simulink library "csu_ctp_coarse_thruster_pulse_command_lib"  (R2014b)
settings: Solver=ode113  StartTime=0.0  StopTime=10.0  RelTol=1e-3
values from neighbouring files (symbols this model uses):
  cac_acs_minimum_coarse_thruster_ontime = 30    [csc_cac_coarse_acs_ctrl_init.m]
  cac_acs_time_gain_x = 20.0    (= 20)    [csc_cac_coarse_acs_ctrl_init.m]
  cac_acs_time_gain_y = 20.0    (= 20)    [csc_cac_coarse_acs_ctrl_init.m]
  cac_acs_time_gain_z = 20.0    (= 20)    [csc_cac_coarse_acs_ctrl_init.m]
  cac_saturation_axial_force = 0*cac_coarse_thruster_force*cosd(15)+4*cac_coarse_thruster_force    [csc_cac_coarse_acs_ctrl_prep.m]
undefined symbols (not defined in the file or in its folder): cac_num_variable, cac_thr_control, cac_thruster_alloc_pad_coarse_x_tq_full_on, cac_thruster_alloc_pad_coarse_x_tq_variable, cac_thruster_alloc_pad_coarse_y_tq_full_on, cac_thruster_alloc_pad_coarse_y_tq_variable, cac_trq_control
libraries: simulink x1
settings Model: Creator=Jim Kaidy  LastModifiedBy=mstewart

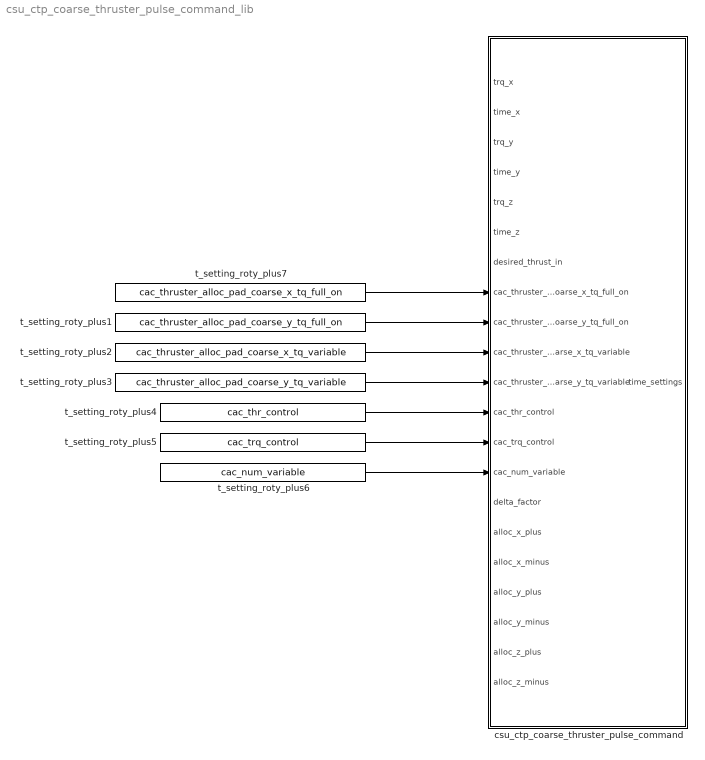
== system csu_ctp_coarse_thruster_pulse_command_lib ==
  csu_ctp_coarse_thruster_pulse_command : Subsystem  TreatAsAtomicUnit=on
  t_setting_roty_plus1 : Constant  Value=cac_thruster_alloc_pad_coarse_y_tq_full_on
  t_setting_roty_plus2 : Constant  Value=cac_thruster_alloc_pad_coarse_x_tq_variable
  t_setting_roty_plus3 : Constant  Value=cac_thruster_alloc_pad_coarse_y_tq_variable
  t_setting_roty_plus4 : Constant  Value=cac_thr_control
  t_setting_roty_plus5 : Constant  Value=cac_trq_control
  t_setting_roty_plus6 : Constant  Value=cac_num_variable
  t_setting_roty_plus7 : Constant  Value=cac_thruster_alloc_pad_coarse_x_tq_full_on
  wires:
  t_setting_roty_plus7/1 -> csu_ctp_coarse_thruster_pulse_command/8(cac_thruster_alloc_pad_coarse_x_tq_full_on)
  t_setting_roty_plus1/1 -> csu_ctp_coarse_thruster_pulse_command/9(cac_thruster_alloc_pad_coarse_y_tq_full_on)
  t_setting_roty_plus2/1 -> csu_ctp_coarse_thruster_pulse_command/10(cac_thruster_alloc_pad_coarse_x_tq_variable)
  t_setting_roty_plus3/1 -> csu_ctp_coarse_thruster_pulse_command/11(cac_thruster_alloc_pad_coarse_y_tq_variable)
  t_setting_roty_plus4/1 -> csu_ctp_coarse_thruster_pulse_command/12(cac_thr_control)
  t_setting_roty_plus5/1 -> csu_ctp_coarse_thruster_pulse_command/13(cac_trq_control)
  t_setting_roty_plus6/1 -> csu_ctp_coarse_thruster_pulse_command/14(cac_num_variable)
  ? -> csu_ctp_coarse_thruster_pulse_command/15(delta_factor)
  ? -> csu_ctp_coarse_thruster_pulse_command/16(alloc_x_plus)
  ? -> csu_ctp_coarse_thruster_pulse_command/17(alloc_x_minus)
  ? -> csu_ctp_coarse_thruster_pulse_command/18(alloc_y_plus)
  ? -> csu_ctp_coarse_thruster_pulse_command/19(alloc_y_minus)
  ? -> csu_ctp_coarse_thruster_pulse_command/20(alloc_z_plus)
  ? -> csu_ctp_coarse_thruster_pulse_command/21(alloc_z_minus)

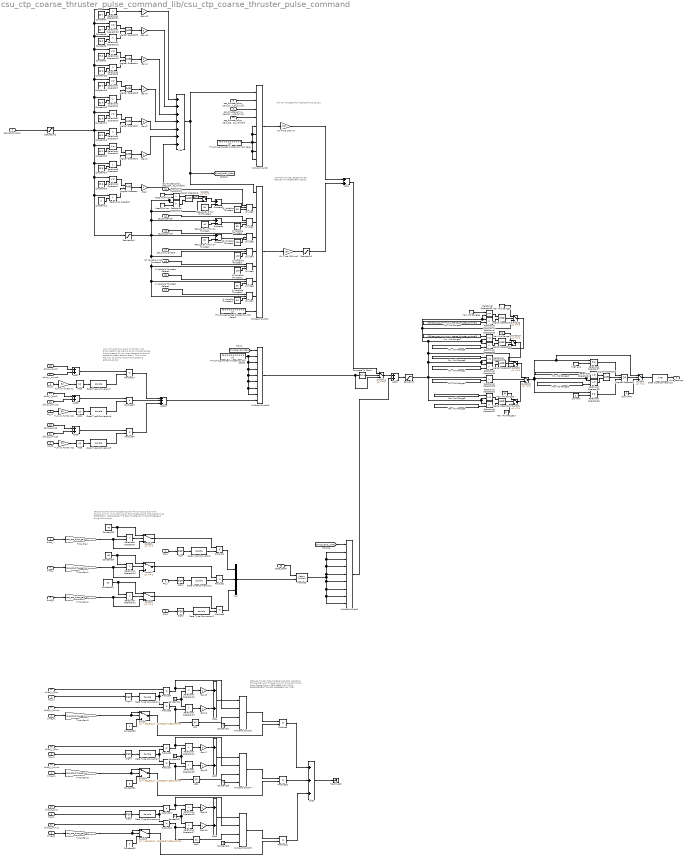
== system csu_ctp_coarse_thruster_pulse_command_lib/csu_ctp_coarse_thruster_pulse_command ==
  note: Attitude Control WItout Descent Control -Coasting
      | Torque Sign and Torque Axis On Time Command
      | From Phase Plane - REPLACED WITH PAIR
      | ENFORCEMENT ON FOR DIFFERENTIAL
      | TIME
  note: Attitude Control With Descent Control Firing
      | Torque Sign and Torque Axis On TIme Command
      | From Phase Plane With Delta Time Offset Matrix (delta_factor)
      | To Bias Thruster On Times Of Descent Firing Commands
  note: Full On Thrusters For Highest Thrust Levels
  note: Variable Thruster Selections For
      |  Desired Thrust Between Levels
  note: ACS with enforcing pairs on for 50 ms
      | to allow delta time logic to allow smaller
      | torque times instead of just when descent
      | control of coarse thrusters asks for them.
      | This is now the way to control biprop and
      | coasting attitude control
  trq_x : Inport
  time_x : Inport  Port=2
  trq_y : Inport  Port=3
  time_y : Inport  Port=4
  trq_z : Inport  Port=5
  time_z : Inport  Port=6
  desired_thrust_in : Inport  Port=7
  cac_thruster_alloc_pad_coarse_x_tq_full_on : Inport  Port=8
  cac_thruster_alloc_pad_coarse_y_tq_full_on : Inport  Port=9
  cac_thruster_alloc_pad_coarse_x_tq_variable : Inport  Port=10
  cac_thruster_alloc_pad_coarse_y_tq_variable : Inport  Port=11
  cac_thr_control : Inport  Port=12
  cac_trq_control : Inport  Port=13
  cac_num_variable : Inport  Port=14
  delta_factor : Inport  Port=15
  alloc_x_plus : Inport  Port=16
  alloc_x_minus : Inport  Port=17
  alloc_y_plus : Inport  Port=18
  alloc_y_minus : Inport  Port=19
  alloc_z_plus : Inport  Port=20
  alloc_z_minus : Inport  Port=21
  "   " : Constant  Value=120
  10 Variable Axial Thrusters1 : InportShadow  Port=13
  10 Variable Thrusters : Constant  Value=100
  10 Variable Thrusters1 : Constant  Value=100
  12 Variable Thrusters : Constant  Value=120
  6 Variable Thrusters : Constant  Value=60
  6 Variable Thrusters Select1 : InportShadow  Port=11
  6 Variable Thrusters1 : Constant  Value=60
  8 Variable Thrusters : Constant  Value=80
  8 Variable Thrusters Select1 : InportShadow  Port=12
  8 Variable Thrusters1 : Constant  Value=80
  Abs{,1..5} (6 alike) : Abs
  Add : Sum  Inputs=+++++++
  Add{1..2,4..9} (8 alike) : Sum
  Add10 : Sum  Inputs=+++
  Add3 : Sum  Inputs=+++
  Compare To Zero1 : simulink/Logic and Bit Operations/Compare To Zero  relop===  OutDataTypeStr=boolean
  Constant1 : Constant  Value=75.2
  Constant{12,21..22,25..28,30..32} (10 alike) : Constant  Value=0
  Constant13 : Constant  Value=23.6
  Constant14 : Constant  Value=23.6
  Constant15 : Constant  Value=42.1
  Constant16 : Constant  Value=42.1
  Constant17 : Constant  Value=51.6
  Constant18 : Constant  Value=51.6
  Constant19 : Constant  Value=65.6
  Constant2 : Constant  Value=75.2
  Constant20 : Constant  Value=65.6
  Constant23 : Constant  Value=40
  Constant24 : Constant  Value=80
  Constant29 : Constant  Value=20
  Constant3 : Constant  Value=93.7
  Constant4 : Constant  Value=93.7
  Data Type Conversion{,1..2,4..9} (9 alike) : DataTypeConversion  OutDataTypeStr=double
  Data Type Conversion3 : DataTypeConversion  OutDataTypeStr=uint8
  Divide{1..7} (7 alike) : Product  Inputs=**/
  Don't Fire : Constant  Value=0
  Gain{,6,8,10} (4 alike) : Gain
  Gain{1,5,7,9} (4 alike) : Gain  Gain=2
  Gain11 : Gain  Gain=6
  Gain12 : Gain  Gain=7
  Gain2 : Gain  Gain=3
  Gain3 : Gain  Gain=4
  Gain4 : Gain  Gain=5
  High end : Constant  Value=100
  Keep Out High : Constant  Value=120
  Keep Out Low : Constant  Value=102
  Logical Operator{,1..7,9..12} (12 alike) : Logic  AllPortsSameDT=off  OutDataTypeStr=boolean
  Logical Operator8 : Logic  Operator=OR  Inputs=3  AllPortsSameDT=off  OutDataTypeStr=boolean
  Low end : Constant  Value=0
  Max Mid Range1 : Constant  Value=70
  Max Mid Range10 : Constant  Value=0
  Max Mid Range2 : Constant  Value=100
  Max Mid Range3 : Constant  Value=cac_acs_minimum_coarse_thruster_ontime
  Max Mid Range4 : Constant  Value=30
  Max Mid Range5 : Constant  Value=cac_acs_minimum_coarse_thruster_ontime
  Max Mid Range6 : Constant  Value=100
  Max Mid Range9 : Constant  Value=cac_acs_minimum_coarse_thruster_ontime/2
  Min  Mid Range1 : Constant  Value=cac_acs_minimum_coarse_thruster_ontime
  Min  Mid Range3 : Constant  Value=100-cac_acs_minimum_coarse_thruster_ontime
  Min  Mid Range4 : Constant  Value=cac_acs_minimum_coarse_thruster_ontime
  Min  Mid Range5 : Constant  Value=100-cac_acs_minimum_coarse_thruster_ontime/2
  Min  Mid Range6 : Constant  Value=100-cac_acs_minimum_coarse_thruster_ontime
  Min  Mid Range7 : Constant  Value=100-cac_acs_minimum_coarse_thruster_ontime/2
  Min  Mid Range8 : Constant  Value=100-cac_acs_minimum_coarse_thruster_ontime
  Multiport Switch{,1..2,6} (4 alike) : MultiPortSwitch  DataPortOrder=Specify indices  Inputs=5  DataPortIndices={7,6,5,4,3,2,1,0}
  Multiport Switch3 : MultiPortSwitch  DataPortOrder=Specify indices  Inputs=5  DataPortIndices={2,1,0}
  Multiport Switch4 : MultiPortSwitch  DataPortOrder=Specify indices  Inputs=5  DataPortIndices={2,1,0}
  Multiport Switch5 : MultiPortSwitch  DataPortOrder=Specify indices  Inputs=5  DataPortIndices={2,1,0}
  Mux : Mux  Inputs=3
  On Time 100 ms : Gain  Gain=100
  On Time 100 ms2 : Gain  Gain=100
  Product{1..4,6..16} (15 alike) : Product
  Product5 : Product  Multiplication=Matrix(*)  RndMeth=Zero
  "Reduce By 2 Full On Thrusters " : Constant  Value=20
  "Reduce By 4 Full On Thrusters " : Constant  Value=40
  Reduce By 6 Full OnThrusters : Constant  Value=60
  Relational Operator{,2,4,6,8,12..17,19,21..23,28,30,32,34,36} (20 alike) : RelationalOperator  Operator=>  OutDataTypeStr=boolean
  Relational Operator{1,3,5,7,18,20} (6 alike) : RelationalOperator  Operator=<=  OutDataTypeStr=boolean
  Relational Operator10 : RelationalOperator  Operator=<  OutDataTypeStr=boolean
  Relational Operator11 : RelationalOperator  Operator=<  OutDataTypeStr=boolean
  Relational Operator{24..25,29,31,33,35} (6 alike) : RelationalOperator  OutDataTypeStr=boolean
  Relational Operator26 : RelationalOperator  Operator===  OutDataTypeStr=boolean
  Relational Operator27 : RelationalOperator  Operator===  OutDataTypeStr=boolean
  Relational Operator9 : RelationalOperator  Operator=<  OutDataTypeStr=boolean
  Saturation : Saturate  UpperLimit=100.0  LowerLimit=0.0
  Saturation1 : Saturate  UpperLimit=100  LowerLimit=0
  Saturation2 : Saturate  UpperLimit=cac_saturation_axial_force  LowerLimit=0
  Saturation3 : Saturate  UpperLimit=120  LowerLimit=0
  Sign{,1..5} (6 alike) : Signum
  Subtract : Sum  Inputs=+-
  Subtract1 : Sum  Inputs=+-
  Subtract2 : Sum  Inputs=+-
  Switch : Switch  Criteria=u2 > Threshold  Threshold=cac_acs_minimum_coarse_thruster_ontime
  Switch{1..3,6..13} (11 alike) : Switch  Criteria=u2 ~= 0
  Switch4 : Switch  Criteria=u2 > Threshold  Threshold=cac_acs_minimum_coarse_thruster_ontime
  Switch5 : Switch  Criteria=u2 > Threshold  Threshold=cac_acs_minimum_coarse_thruster_ontime
  Terminator : Terminator
  Thrust Augmented Allocations Null Case : Constant  Value=[0 0 0 0 0 0 0 0 0 0 0 0]'  VectorParams1D=off
  Thrust Augmented Allocations Null Case1 : Constant  Value=[0 0 0 0 0 0 0 0 0 0 0 0]'  VectorParams1D=off
  Thrust Augmented Allocations Null Case2 : Constant  Value=[0 0 0 0 0 0 0 0 0 0 0 0]'  VectorParams1D=off
  Time Gain : Gain  Gain=cac_acs_time_gain_x
  Time Gain1 : Gain  Gain=cac_acs_time_gain_y
  Time Gain2 : Gain  Gain=cac_acs_time_gain_z
  Time Gain3 : Gain  Gain=cac_acs_time_gain_x
  Time Gain4 : Gain  Gain=cac_acs_time_gain_z
  Time Gain5 : Gain  Gain=cac_acs_time_gain_y
  Turn on for 50 ms : Gain  Gain=50
  Turn on for 50 ms1 : Gain  Gain=50
  Turn on for 50 ms2 : Gain  Gain=50
  alloc_x_minus1 : InportShadow  Port=17
  alloc_x_plus1 : InportShadow  Port=16
  alloc_y_minus1 : InportShadow  Port=19
  alloc_y_plus1 : InportShadow  Port=18
  alloc_z_minus2 : InportShadow  Port=21
  alloc_z_plus2 : InportShadow  Port=20
  time_x1 : InportShadow  Port=2
  time_y1 : InportShadow  Port=4
  time_z1 : InportShadow  Port=6
  trq_x1 : InportShadow
  trq_x2 : InportShadow
  trq_y1 : InportShadow  Port=3
  trq_y2 : InportShadow  Port=3
  trq_z1 : InportShadow  Port=5
  trq_z3 : InportShadow  Port=5
  time_settings : Outport
  wires:
  Data Type Conversion3/1 -> time_settings/1
  trq_x/1 -> Sign/1
  time_x/1 -> Time Gain/1
  desired_thrust_in/1 -> Saturation2/1
  Constant12/1 -> Relational Operator/2
  Constant13/1 -> Relational Operator1/2
  Relational Operator1/1 -> Logical Operator/1
  Relational Operator/1 -> Logical Operator/2
  Constant14/1 -> Relational Operator2/2
  Constant15/1 -> Relational Operator3/2
  Relational Operator3/1 -> Logical Operator1/1
  Relational Operator2/1 -> Logical Operator1/2
  Constant16/1 -> Relational Operator4/2
  Constant17/1 -> Relational Operator5/2
  Relational Operator5/1 -> Logical Operator2/1
  Relational Operator4/1 -> Logical Operator2/2
  Constant18/1 -> Relational Operator6/2
  Constant19/1 -> Relational Operator7/2
  Relational Operator7/1 -> Logical Operator3/1
  Relational Operator6/1 -> Logical Operator3/2
  Constant20/1 -> Relational Operator8/2
  Logical Operator/1 -> Gain/1
  Logical Operator1/1 -> Gain1/1
  Logical Operator2/1 -> Gain2/1
  Logical Operator3/1 -> Gain3/1
  Gain4/1 -> Add/3
  Gain3/1 -> Add/4
  Gain2/1 -> Add/5
  Gain1/1 -> Add/6
  Gain/1 -> Add/7
  Add/1 -> [thrust_level_index], Multiport Switch1/1, Multiport Switch/1
  "Reduce By 2 Full On Thrusters "/1 -> Subtract/2
  "Reduce By 4 Full On Thrusters "/1 -> Subtract1/2
  Reduce By 6 Full OnThrusters/1 -> Subtract2/2
  Subtract2/1 -> Divide2/2  "Less 6 Thrusters"
  Multiport Switch/1 -> On Time 100 ms/1
  Multiport Switch1/1 -> On Time 100 ms2/1  "Residual Thrust"
  On Time 100 ms/1 -> Add1/1  "Full On Thrusters"
  Time Gain/1 -> Switch1/3, Relational Operator9/2
  Time Gain1/1 -> Switch2/3, Relational Operator10/2
  Time Gain2/1 -> Switch3/3, Relational Operator11/2
  Relational Operator9/1 -> Switch1/2
  Constant23/1 -> Relational Operator9/1, Switch1/1
  Constant24/1 -> Relational Operator10/1, Switch2/1
  Constant29/1 -> Relational Operator11/1, Switch3/1
  Relational Operator10/1 -> Switch2/2
  Relational Operator11/1 -> Switch3/2
  Sign/1 -> Data Type Conversion/1
  Data Type Conversion/1 -> Product1/2
  Switch1/1 -> Product1/1
  trq_y/1 -> Sign1/1
  Sign1/1 -> Data Type Conversion1/1
  Data Type Conversion1/1 -> Product2/2
  trq_z/1 -> Sign2/1
  Sign2/1 -> Data Type Conversion2/1
  Data Type Conversion2/1 -> Product3/2
  Switch3/1 -> Product3/1
  delta_factor/1 -> Product5/1
  Add1/1 -> Switch11/1  "Combined Torque Neutral Axial On Times"
  Multiport Switch2/1 -> Add2/2  "Delta Time Settings"
  Add2/1 -> Saturation/1
  Thrust Augmented Allocations Null Case/1 -> Multiport Switch/5, Multiport Switch/6, Multiport Switch/8, Multiport Switch/9, Multiport Switch/7
  Product1/1 -> Mux/1
  Product2/1 -> Mux/2
  Product3/1 -> Mux/3
  Mux/1 -> Product5/2  "Time Settings Torque Command"
  trq_x1/1 -> Sign3/1
  Product5/1 -> Multiport Switch2/9, Multiport Switch2/8, Multiport Switch2/7, Multiport Switch2/6, Multiport Switch2/4, Multiport Switch2/3, Multiport Switch2/2, Multiport Switch2/5  "Delta Time Settings"
  [thrust_level_index] -> Multiport Switch2/1
  Sign3/1 -> Data Type Conversion4/1
  alloc_x_plus/1 -> Product4/1
  Data Type Conversion4/1 -> Product4/2, Product8/1
  alloc_x_minus/1 -> Product8/2
  Constant21/1 -> Relational Operator12/2, Relational Operator13/1
  Product4/1 -> Relational Operator12/1, Multiport Switch3/2
  Product8/1 -> Relational Operator13/2, Abs/1
  Gain5/1 -> Add4/1
  Gain6/1 -> Add4/2
  Add4/1 -> Multiport Switch3/1
  Relational Operator12/1 -> Gain5/1
  Relational Operator13/1 -> Gain6/1
  Constant22/1 -> Multiport Switch3/4
  Product9/1 -> Add3/1
  Switch/1 -> Product9/2
  Multiport Switch3/1 -> Product9/1
  trq_y1/1 -> Sign4/1
  Sign4/1 -> Data Type Conversion5/1
  alloc_y_plus/1 -> Product6/1
  Data Type Conversion5/1 -> Product7/1, Product6/2
  Constant25/1 -> Relational Operator15/1, Relational Operator14/2
  Product6/1 -> Multiport Switch4/2, Relational Operator14/1
  Product7/1 -> Abs1/1, Relational Operator15/2
  Gain7/1 -> Add5/1
  Gain8/1 -> Add5/2
  Add5/1 -> Multiport Switch4/1
  Relational Operator14/1 -> Gain7/1
  Relational Operator15/1 -> Gain8/1
  Constant26/1 -> Multiport Switch4/4
  Switch4/1 -> Product10/2
  Multiport Switch4/1 -> Product10/1
  Product10/1 -> Add3/2
  Sign5/1 -> Data Type Conversion6/1
  Data Type Conversion6/1 -> Product12/2, Product13/1
  alloc_z_minus/1 -> Product13/2
  Constant27/1 -> Relational Operator16/2, Relational Operator17/1
  Product12/1 -> Relational Operator16/1, Multiport Switch5/2
  Product13/1 -> Relational Operator17/2, Abs2/1
  Gain9/1 -> Add6/1
  Gain10/1 -> Add6/2
  Add6/1 -> Multiport Switch5/1
  Relational Operator16/1 -> Gain9/1
  Relational Operator17/1 -> Gain10/1
  Constant28/1 -> Multiport Switch5/4
  Switch5/1 -> Product11/2
  Multiport Switch5/1 -> Product11/1
  Product11/1 -> Add3/3
  trq_z1/1 -> Sign5/1
  alloc_z_plus/1 -> Product12/1
  alloc_y_minus/1 -> Product7/2
  Abs/1 -> Multiport Switch3/3
  Abs1/1 -> Multiport Switch4/3
  Abs2/1 -> Multiport Switch5/3
  time_x1/1 -> Time Gain3/1
  Constant30/1 -> Switch/3
  time_y1/1 -> Time Gain5/1
  Constant31/1 -> Switch4/3
  time_z1/1 -> Time Gain4/1
  Constant32/1 -> Switch5/3
  Time Gain3/1 -> Switch/2, Switch/1
  Time Gain5/1 -> Switch4/1, Switch4/2
  Time Gain4/1 -> Switch5/2, Switch5/1
  Constant1/1 -> Relational Operator18/2
  Constant2/1 -> Relational Operator19/2
  Constant3/1 -> Relational Operator20/2
  Saturation2/1 -> Saturation3/1, Relational Operator/1, Relational Operator1/1, Relational Operator2/1, Relational Operator3/1, Relational Operator6/1, Relational Operator18/1, Relational Operator21/1, Relational Operator20/1, Relational Operator19/1, Relational Operator8/1, Relational Operator7/1, Relational Operator5/1, Relational Operator4/1
  Constant4/1 -> Relational Operator21/2
  cac_thruster_alloc_pad_coarse_x_tq_full_on/1 -> Multiport Switch/2
  cac_thruster_alloc_pad_coarse_y_tq_full_on/1 -> Multiport Switch/3
  cac_thruster_alloc_pad_coarse_x_tq_variable/1 -> Multiport Switch/4
  Relational Operator18/1 -> Logical Operator4/1
  Relational Operator8/1 -> Logical Operator4/2
  Logical Operator4/1 -> Gain4/1
  Relational Operator20/1 -> Logical Operator5/1
  Relational Operator19/1 -> Logical Operator5/2
  Logical Operator5/1 -> Gain11/1
  Relational Operator21/1 -> Gain12/1
  Gain11/1 -> Add/2
  Gain12/1 -> Add/1
  On Time 100 ms2/1 -> Saturation1/1  "Variable Time"
  6 Variable Thrusters/1 -> Divide2/3
  Divide2/1 -> Multiport Switch1/2
  cac_thruster_alloc_pad_coarse_y_tq_variable/1 -> Divide2/1
  cac_thr_control/1 -> Divide1/1
  8 Variable Thrusters/1 -> Divide1/3
  Subtract1/1 -> Divide1/2  "Less 4 Thrusters"
  Divide3/1 -> Multiport Switch1/4
  cac_trq_control/1 -> Divide3/1
  Subtract/1 -> Divide3/2  "Less 2 Thrusters"
  10 Variable Thrusters/1 -> Divide3/3
  Divide4/1 -> Multiport Switch1/5
  cac_num_variable/1 -> Divide4/1
  12 Variable Thrusters/1 -> Divide4/3
  Divide5/1 -> Multiport Switch1/6
  10 Variable Thrusters1/1 -> Divide5/3
  10 Variable Axial Thrusters1/1 -> Divide5/1
  Divide6/1 -> Multiport Switch1/7
  8 Variable Thrusters1/1 -> Divide6/3
  8 Variable Thrusters Select1/1 -> Divide6/1
  Divide7/1 -> Multiport Switch1/8
  6 Variable Thrusters1/1 -> Divide7/3
  6 Variable Thrusters Select1/1 -> Divide7/1
  Thrust Augmented Allocations Null Case1/1 -> Multiport Switch1/9
  Add3/1 -> Terminator/1  "Coast ACS"
  Saturation1/1 -> Add1/2
  Divide1/1 -> Multiport Switch1/3
  Saturation3/1 -> Subtract/1, Relational Operator23/1, Relational Operator22/2, Switch6/3, Subtract1/1, Divide7/2, Divide6/2, Divide5/2, Divide4/2
  Keep Out High/1 -> Relational Operator22/1
  Relational Operator22/1 -> Logical Operator6/1
  Keep Out Low/1 -> Relational Operator23/2
  Relational Operator23/1 -> Logical Operator6/2
  Logical Operator6/1 -> Switch6/2
  "   "/1 -> Switch6/1
  Switch6/1 -> Subtract2/1
  Relational Operator24/1 -> Logical Operator7/1
  Relational Operator25/1 -> Logical Operator7/2
  Min  Mid Range3/1 -> Relational Operator24/1
  Max Mid Range5/1 -> Relational Operator25/2
  High end/1 -> Relational Operator27/2
  Relational Operator27/1 -> Logical Operator8/1
  Logical Operator7/1 -> Logical Operator8/2
  Relational Operator26/1 -> Logical Operator8/3
  Low end/1 -> Relational Operator26/2
  Switch7/1 -> Data Type Conversion3/1
  Logical Operator8/1 -> Switch7/2
  Don't Fire/1 -> Switch7/3
  Min  Mid Range6/1 -> Relational Operator29/1
  Min  Mid Range1/1 -> Relational Operator30/2
  Relational Operator29/1 -> Logical Operator9/1
  Relational Operator30/1 -> Logical Operator9/2
  Max Mid Range3/1 -> Relational Operator31/1
  Max Mid Range9/1 -> Relational Operator32/2
  Relational Operator31/1 -> Logical Operator10/1
  Relational Operator32/1 -> Logical Operator10/2
  Logical Operator10/1 -> Switch9/2
  Max Mid Range4/1 -> Switch9/1
  Logical Operator9/1 -> Switch8/2
  Switch9/1 -> Switch10/3
  Switch10/1 -> Relational Operator25/1, Relational Operator24/2, Switch7/1, Relational Operator27/1, Relational Operator26/1
  alloc_x_plus1/1 -> Add7/1
  alloc_x_minus1/1 -> Add7/2
  Abs3/1 -> Data Type Conversion7/1
  trq_x2/1 -> Turn on for 50 ms/1
  Add7/1 -> Product14/1
  Data Type Conversion7/1 -> Product14/2
  Turn on for 50 ms/1 -> Abs3/1
  alloc_y_plus1/1 -> Add8/1
  alloc_y_minus1/1 -> Add8/2
  Abs4/1 -> Data Type Conversion8/1
  Add8/1 -> Product15/1
  Data Type Conversion8/1 -> Product15/2
  Turn on for 50 ms1/1 -> Abs4/1
  trq_y2/1 -> Turn on for 50 ms1/1
  Product14/1 -> Add10/1
  Product15/1 -> Add10/2
  [thrust_level_index] -> Multiport Switch6/1
  Multiport Switch6/1 -> Switch11/3, Compare To Zero1/1  "For ACS Turn On Both and Use Deltas to Reduce Times For Better Than 30 ms Minimum On TImes"
  Compare To Zero1/1 -> Switch11/2
  Switch11/1 -> Add2/1
  Switch2/1 -> Product2/1
  time_y/1 -> Time Gain1/1
  time_z/1 -> Time Gain2/1
  Min  Mid Range4/1 -> Relational Operator28/2
  Relational Operator28/1 -> Switch10/2
  Switch8/1 -> Switch10/1
  Max Mid Range6/1 -> Relational Operator33/1
  Min  Mid Range5/1 -> Relational Operator34/2
  Min  Mid Range7/1 -> Relational Operator35/1
  Min  Mid Range8/1 -> Relational Operator36/2
  Saturation/1 -> Relational Operator35/2, Relational Operator36/1, Switch12/3, Relational Operator34/1, Relational Operator33/2, Switch8/1, Relational Operator29/2, Relational Operator30/1, Relational Operator28/1, Relational Operator32/1, Relational Operator31/2
  Relational Operator33/1 -> Logical Operator11/1
  Relational Operator34/1 -> Logical Operator11/2
  Logical Operator11/1 -> Switch12/2
  Max Mid Range2/1 -> Switch12/1
  Relational Operator35/1 -> Logical Operator12/1
  Relational Operator36/1 -> Logical Operator12/2
  Logical Operator12/1 -> Switch13/2
  Max Mid Range1/1 -> Switch13/1
  Switch13/1 -> Switch8/3
  Switch12/1 -> Switch13/3
  Max Mid Range10/1 -> Switch9/3
  Thrust Augmented Allocations Null Case2/1 -> Multiport Switch6/3, Multiport Switch6/4, Multiport Switch6/5, Multiport Switch6/6, Multiport Switch6/7, Multiport Switch6/8, Multiport Switch6/2
  Add10/1 -> Multiport Switch6/9
  alloc_z_plus2/1 -> Add9/1
  Abs5/1 -> Data Type Conversion9/1
  Add9/1 -> Product16/1
  Data Type Conversion9/1 -> Product16/2
  Turn on for 50 ms2/1 -> Abs5/1
  alloc_z_minus2/1 -> Add9/2
  trq_z3/1 -> Turn on for 50 ms2/1
  Product16/1 -> Add10/3
